simulink model "COM_BancMonitor"  (Simulink 8.6)
settings: Solver=FixedStepDiscrete  StartTime=0.0  StopTime=inf  FixedStep=ComMinSampleTime  RelTol=1e-3
values from neighbouring files (symbols this model uses):
  ComMinSampleTime = 1/400    (= 0.0025)    [init_BancMonitor.m]
  g = 9.81    [init_BancMonitor.m]
  LandingHeight = 0.08    [init_BancMonitor.m]
  Ts_AttitudeLoop = 1/200    (= 0.005)    [init_BancMonitor.m]
  Ts_PositionLoop = 1/100    (= 0.01)    [init_BancMonitor.m]
undefined symbols (not defined in the file or in its folder): a_PWM, b_PWM, BiasAcc, DiscIntNeverNeededParam, Gumstix, m, MaxThrottle, MinThrottle, MPU6050, PositionSecuMax, PositionSecuMin, Tacc, time_unfolding, Tmax, Tmin, TorquesSat, UAVstruct
undefined symbols (not defined in the file): AccMax, AccMaxScenario, AccMin, AccMinScenario, b_est0, dc_open, PositionMax, PositionMin, SpeedMax, SpeedMaxScenario, SpeedMin, SpeedMinScenario, Ts_detector, Ts_Wifi
libraries: simulink x34, custom_lib x27, simulink_extras x11
(part 3 of 3)

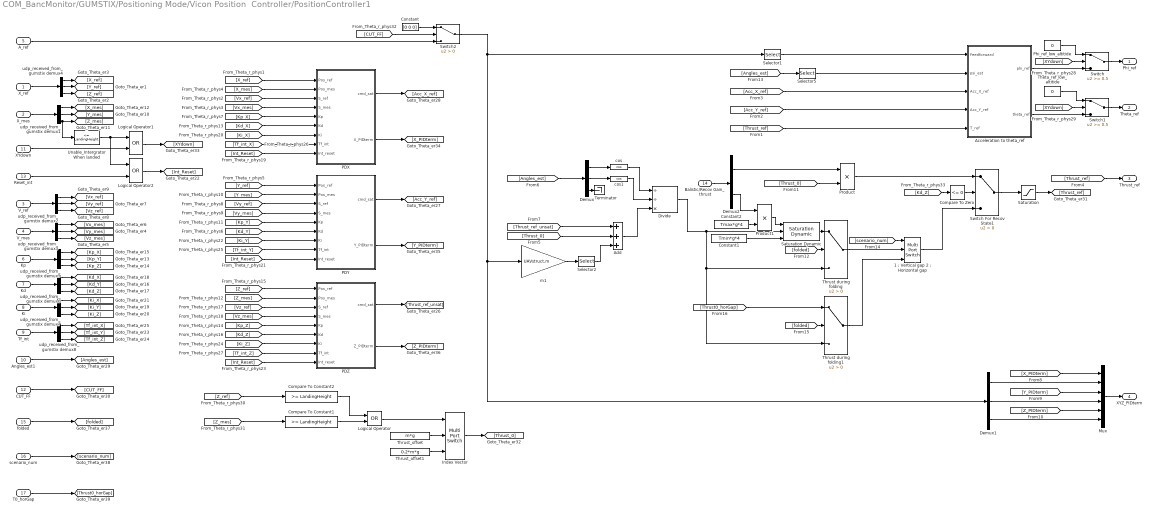
== system COM_BancMonitor/GUMSTIX/Positioning Mode/Vicon Position  Controller/PositionController1 ==
  X_ref : Inport
  X_mes : Inport  Port=2
  V_ref : Inport  Port=3
  V_mes : Inport  Port=4
  A_ref : Inport  Port=5
  Kp : Inport  Port=6
  Kd : Inport  Port=7
  Ki : Inport  Port=8
  Tf_int : Inport  Port=9
  Angles_est1 : Inport  Port=10
  XYdown : Inport  Port=11
  CUT_FF : Inport  Port=12
  Reset_int : Inport  Port=13
  Balistic/Recov Gain_thrust : Inport  Port=14
  folded : Inport  Port=15
  scenario_num : Inport  Port=16
  T0_horGap : Inport  Port=17
  "1 : Vertical gap 2 : Horizontal gap" : MultiPortSwitch  Inputs=2
  Acceleration to theta_ref : Subsystem
  Add : Sum  Inputs=+++
  Compare To Constant1 : simulink/Logic and Bit Operations/Compare To Constant  relop=>=  const=LandingHeight  OutDataTypeStr=uint8
  Compare To Constant2 : simulink/Logic and Bit Operations/Compare To Constant  relop=>=  const=LandingHeight  OutDataTypeStr=uint8
  Compare To Zero : simulink/Logic and Bit Operations/Compare To Zero  relop=<=  OutDataTypeStr=boolean
  Constant : Constant  Value=[0 0 0]  OutDataTypeStr=Inherit: Inherit via back propagation
  Constant1 : Constant  Value=Tmin*g*4  OutDataTypeStr=Inherit: Inherit via back propagation
  Constant2 : Constant  Value=Tmax*g*4  OutDataTypeStr=Inherit: Inherit via back propagation
  Demux : Demux  Outputs=3
  Demux1 : Demux  Outputs=3
  Demux2 : Demux  Outputs=2
  Divide : Product  Inputs=//*
  Index Vector : MultiPortSwitch  Inputs=2  DiagnosticForDefault=None
  Logical Operator : Logic  Operator=OR  AllPortsSameDT=off  OutDataTypeStr=boolean
  Logical Operator1 : Logic  Operator=OR  AllPortsSameDT=off  OutDataTypeStr=boolean
  Logical Operator2 : Logic  Operator=OR  AllPortsSameDT=off  OutDataTypeStr=boolean
  Mux : Mux  Inputs=[5 1 5 1 5 1]
  PDX : Subsystem  mask{Max_Sat=20*pi/180*9.81, Min_Sat=-20*pi/180*9.81}
  PDY : Subsystem  mask{Max_Sat=20*pi/180*9.81, Min_Sat=-20*pi/180*9.81}
  PDZ : Subsystem  mask{Max_Sat=Tmax*g*4, Min_Sat=Tmin*g*4}
  Phi_ref_low_altitide : Constant  Value=0  OutDataTypeStr=Inherit: Inherit via back propagation
  Product : Product
  Product1 : Product
  Saturation : Saturate  UpperLimit=Tmax*g*4  LowerLimit=Tmin*g*4
  Saturation Dynamic : simulink/Discontinuities/Saturation Dynamic  OutMin=[]  OutMax=[]  OutDataTypeStr=Inherit: Same as second input  OutDataType=fixdt(1, 16)  OutScaling=2^-10  DoSatur=off
  Selector1 : Selector  InputPortWidth=3  IndexOptions=Index vector (dialog)  Indices=[1 2]  OutputSizes=1
  Selector2 : Selector  InputPortWidth=3  IndexOptions=Index vector (dialog)  Indices=[3]  OutputSizes=1
  Selector5 : Selector  InputPortWidth=3  IndexOptions=Index vector (dialog)  Indices=[3]  OutputSizes=1
  Switch : Switch  Threshold=0.5
  Switch For Recov State1 : Switch  Criteria=u2 > Threshold
  Switch1 : Switch  Threshold=0.5
  Switch2 : Switch  Criteria=u2 > Threshold
  Terminator : Terminator
  Theta_ref_low_altitide : Constant  Value=0  OutDataTypeStr=Inherit: Inherit via back propagation
  Thrust during folding : Switch  Criteria=u2 > Threshold
  Thrust during folding1 : Switch  Criteria=u2 > Threshold
  Thrust_offset : Constant  Value=m*g  OutDataTypeStr=single  SampleTime=-1
  Thrust_offset1 : Constant  Value=0.2*m*g  OutDataTypeStr=single  SampleTime=-1
  Unable_Intergrator When landed : simulink/Logic and Bit Operations/Compare To Constant  relop=<=  const=LandingHeight  OutDataTypeStr=uint8
  cos : Trigonometry  Operator=cos
  cos1 : Trigonometry  Operator=cos
  m1 : Gain  Gain=UAVstruct.m
  udp_received_from_gumstix demux{1..8} (8 alike) : Demux  Outputs=[1 1 1]
  Phi_ref : Outport
  Theta_ref : Outport  Port=2
  Thrust_ref : Outport  Port=3
  XYZ_PIDterm : Outport  Port=4
  wires:
  udp_received_from_gumstix demux3/3 -> [Vz_mes]
  udp_received_from_gumstix demux3/2 -> [Vy_mes]
  udp_received_from_gumstix demux3/1 -> [Vx_mes]
  V_mes/1 -> udp_received_from_gumstix demux3/1
  udp_received_from_gumstix demux4/1 -> [X_ref]
  udp_received_from_gumstix demux4/2 -> [Y_ref]
  X_mes/1 -> udp_received_from_gumstix demux1/1
  udp_received_from_gumstix demux1/1 -> [X_mes]
  udp_received_from_gumstix demux1/2 -> [Y_mes]
  udp_received_from_gumstix demux1/3 -> [Z_mes], Unable_Intergrator When landed/1
  udp_received_from_gumstix demux2/3 -> [Vz_ref]
  udp_received_from_gumstix demux2/2 -> [Vy_ref]
  udp_received_from_gumstix demux2/1 -> [Vx_ref]
  V_ref/1 -> udp_received_from_gumstix demux2/1
  Kp/1 -> udp_received_from_gumstix demux5/1
  udp_received_from_gumstix demux5/3 -> [Kp_Z]
  udp_received_from_gumstix demux5/2 -> [Kp_Y]
  udp_received_from_gumstix demux5/1 -> [Kp_X]
  Kd/1 -> udp_received_from_gumstix demux6/1
  udp_received_from_gumstix demux6/3 -> [Kd_Z]
  udp_received_from_gumstix demux6/2 -> [Kd_Y]
  udp_received_from_gumstix demux6/1 -> [Kd_X]
  udp_received_from_gumstix demux4/3 -> [Z_ref]
  udp_received_from_gumstix demux7/3 -> [Ki_Z]
  udp_received_from_gumstix demux7/2 -> [Ki_Y]
  udp_received_from_gumstix demux7/1 -> [Ki_X]
  Ki/1 -> udp_received_from_gumstix demux7/1
  udp_received_from_gumstix demux8/3 -> [Tf_int_Z]
  udp_received_from_gumstix demux8/2 -> [Tf_int_Y]
  udp_received_from_gumstix demux8/1 -> [Tf_int_X]
  Tf_int/1 -> udp_received_from_gumstix demux8/1
  Acceleration to theta_ref/1(phi_ref) -> Switch/3
  [XYdown] -> Switch/2
  [XYdown] -> Switch1/2
  Acceleration to theta_ref/2(theta_ref) -> Switch1/3
  Switch1/1 -> Theta_ref/1
  Switch/1 -> Phi_ref/1
  Phi_ref_low_altitide/1 -> Switch/1
  Theta_ref_low_altitide/1 -> Switch1/1
  [Acc_X_ref] -> Acceleration to theta_ref/3(Acc_X_ref)
  [Acc_Y_ref] -> Acceleration to theta_ref/4(Acc_Y_ref)
  [Thrust_ref] -> Thrust_ref/1
  [Thrust_ref] -> Acceleration to theta_ref/5(T_ref)
  Selector5/1 -> Acceleration to theta_ref/2(psi_est)
  [Angles_est] -> Selector5/1
  Angles_est1/1 -> [Angles_est]
  [Thrust_0] -> Add/2
  [Angles_est] -> Demux/1
  Demux/3 -> Terminator/1
  Demux/1 -> cos/1
  Demux/2 -> cos1/1
  cos/1 -> Divide/1
  cos1/1 -> Divide/2
  [Thrust_ref_unsat] -> Add/1
  Add/1 -> Divide/3
  Selector2/1 -> Add/3
  Selector1/1 -> Acceleration to theta_ref/1(Feedforward)
  Saturation/1 -> [Thrust_ref]
  X_ref/1 -> udp_received_from_gumstix demux4/1
  m1/1 -> Selector2/1
  Thrust_offset/1 -> Index Vector/2
  Thrust_offset1/1 -> Index Vector/3
  Logical Operator/1 -> Index Vector/1
  Compare To Constant1/1 -> Logical Operator/2
  Compare To Constant2/1 -> Logical Operator/1
  [Z_mes] -> Compare To Constant1/1
  [Z_ref] -> Compare To Constant2/1
  Index Vector/1 -> [Thrust_0]
  Unable_Intergrator When landed/1 -> Logical Operator2/1, Logical Operator1/1
  XYdown/1 -> Logical Operator1/2
  Logical Operator1/1 -> [XYdown]
  CUT_FF/1 -> [CUT_FF]
  [CUT_FF] -> Switch2/2
  A_ref/1 -> Switch2/3
  Switch2/1 -> Selector1/1, Demux1/1, m1/1
  Constant/1 -> Switch2/1
  Logical Operator2/1 -> [Int_Reset]
  Reset_int/1 -> Logical Operator2/2
  [X_ref] -> PDX/1(Pos_ref)
  [X_mes] -> PDX/2(Pos_mes)
  [Kp_X] -> PDX/5(Kp)
  [Kd_X] -> PDX/6(Kd)
  [Vx_mes] -> PDX/4(S_mes)
  [Y_ref] -> PDY/1(Pos_ref)
  [Y_mes] -> PDY/2(Pos_mes)
  [Kp_Y] -> PDY/5(Kp)
  [Kd_Y] -> PDY/6(Kd)
  [Vy_ref] -> PDY/3(S_ref)
  [Vy_mes] -> PDY/4(S_mes)
  [Vx_ref] -> PDX/3(S_ref)
  [Ki_X] -> PDX/7(Ki)
  [Ki_Y] -> PDY/7(Ki)
  [Int_Reset] -> PDY/9(Int_reset)
  [Z_ref] -> PDZ/1(Pos_ref)
  [Z_mes] -> PDZ/2(Pos_mes)
  [Vz_ref] -> PDZ/3(S_ref)
  [Vz_mes] -> PDZ/4(S_mes)
  [Kp_Z] -> PDZ/5(Kp)
  [Kd_Z] -> PDZ/6(Kd)
  [Ki_Z] -> PDZ/7(Ki)
  [Tf_int_Y] -> PDY/8(Tf_int)
  [Tf_int_X] -> PDX/8(Tf_int)
  [Int_Reset] -> PDX/9(Int_reset)
  [Tf_int_Z] -> PDZ/8(Tf_int)
  [Int_Reset] -> PDZ/9(Int_reset)
  PDY/1(cmd_sat) -> [Acc_Y_ref]
  PDX/1(cmd_sat) -> [Acc_X_ref]
  PDZ/1(cmd_sat) -> [Thrust_ref_unsat]
  PDX/2(X_PIDterm) -> [X_PIDterm]
  PDY/2(Y_PIDterm) -> [Y_PIDterm]
  PDZ/2(Z_PIDterm) -> [Z_PIDterm]
  [Y_PIDterm] -> Mux/3
  Mux/1 -> XYZ_PIDterm/1
  [X_PIDterm] -> Mux/1
  [Z_PIDterm] -> Mux/5
  [Kd_Z] -> Compare To Zero/1
  Compare To Zero/1 -> Switch For Recov State1/2
  Switch For Recov State1/1 -> Saturation/1
  [Thrust_0] -> Product/2
  Product/1 -> Switch For Recov State1/1
  Demux1/1 -> Mux/2
  Demux1/2 -> Mux/4
  Demux1/3 -> Mux/6
  folded/1 -> [folded]
  [folded] -> Thrust during folding/2
  Saturation Dynamic/1 -> Thrust during folding/1
  Divide/1 -> Saturation Dynamic/2, Thrust during folding1/3, Thrust during folding/3
  Constant1/1 -> Saturation Dynamic/3
  Product1/1 -> Saturation Dynamic/1
  Constant2/1 -> Product1/2
  Balistic/Recov Gain_thrust/1 -> Demux2/1
  Demux2/1 -> Product/1
  Demux2/2 -> Product1/1
  scenario_num/1 -> [scenario_num]
  Thrust during folding/1 -> "1 : Vertical gap 2 : Horizontal gap"/2
  [folded] -> Thrust during folding1/2
  "1 : Vertical gap 2 : Horizontal gap"/1 -> Switch For Recov State1/3
  T0_horGap/1 -> [Thrust0_horGap]
  [Thrust0_horGap] -> Thrust during folding1/1
  Thrust during folding1/1 -> "1 : Vertical gap 2 : Horizontal gap"/3
  [scenario_num] -> "1 : Vertical gap 2 : Horizontal gap"/1

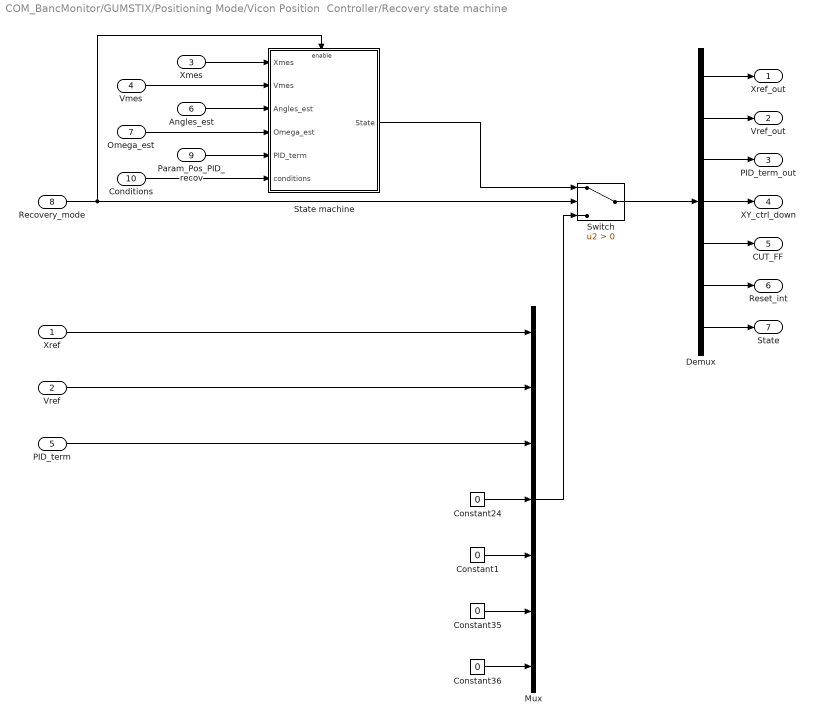
== system COM_BancMonitor/GUMSTIX/Positioning Mode/Vicon Position  Controller/Recovery state machine ==
  Xref : Inport
  Vref : Inport  Port=2
  Xmes : Inport  Port=3
  Vmes : Inport  Port=4
  PID_term : Inport  Port=5
  Angles_est : Inport  Port=6
  Omega_est : Inport  Port=7
  Recovery_mode : Inport  Port=8
  Param_Pos_PID_recov : Inport  Port=9
  Conditions : Inport  Port=10
  Constant{1,24,35..36} (4 alike) : Constant  Value=0  OutDataTypeStr=Inherit: Inherit via back propagation
  Demux : Demux  Outputs=[3 3 12 1 1 1 1]
  Mux : Mux  Inputs=7
  State machine : Subsystem
  Switch : Switch  Criteria=u2 > Threshold
  Xref_out : Outport
  Vref_out : Outport  Port=2
  PID_term_out : Outport  Port=3
  XY_ctrl_down : Outport  Port=4
  CUT_FF : Outport  Port=5
  Reset_int : Outport  Port=6
  State : Outport  Port=7
  wires:
  Demux/1 -> Xref_out/1
  Demux/2 -> Vref_out/1
  Demux/3 -> PID_term_out/1
  Demux/4 -> XY_ctrl_down/1
  Demux/5 -> CUT_FF/1
  Xref/1 -> Mux/1
  Vref/1 -> Mux/2
  Constant24/1 -> Mux/4
  Constant1/1 -> Mux/5
  Mux/1 -> Switch/3
  Vmes/1 -> State machine/2(Vmes)
  Demux/6 -> Reset_int/1
  Constant35/1 -> Mux/6
  PID_term/1 -> Mux/3
  Switch/1 -> Demux/1
  Demux/7 -> State/1
  Constant36/1 -> Mux/7
  Recovery_mode/1 -> Switch/2, State machine/Enable
  State machine/1(State) -> Switch/1
  Angles_est/1 -> State machine/3(Angles_est)
  Omega_est/1 -> State machine/4(Omega_est)
  Xmes/1 -> State machine/1(Xmes)
  Conditions/1 -> State machine/6(conditions)
  Param_Pos_PID_recov/1 -> State machine/5(PID_term)

== system COM_BancMonitor/GUMSTIX/Attitude controller/CTL_ATT_NL/Angles Disturbances/Triggered Subsystem ==
  AnglesDist Mag : Inport
  Dt : Inport  Port=2
  Enable : EnablePort  StatesWhenEnabling=reset
  Constant : Constant  OutDataTypeStr=single
  Discrete-Time Integrator : DiscreteIntegrator  SampleTime=-1  ICPrevOutput=DiscIntNeverNeededParam  ICPrevScaledInput=DiscIntNeverNeededParam
  MATLAB Function : MATLAB Function  TreatAsAtomicUnit=on
  DisturbAngles : Outport  InitialOutput=[0 0 0]
  wires:
  AnglesDist Mag/1 -> MATLAB Function/1(AnglesDistMag)
  Constant/1 -> Discrete-Time Integrator/1
  Discrete-Time Integrator/1 -> MATLAB Function/2(Time)
  Dt/1 -> MATLAB Function/3(Dt)
  MATLAB Function/1(AnglesDist) -> DisturbAngles/1

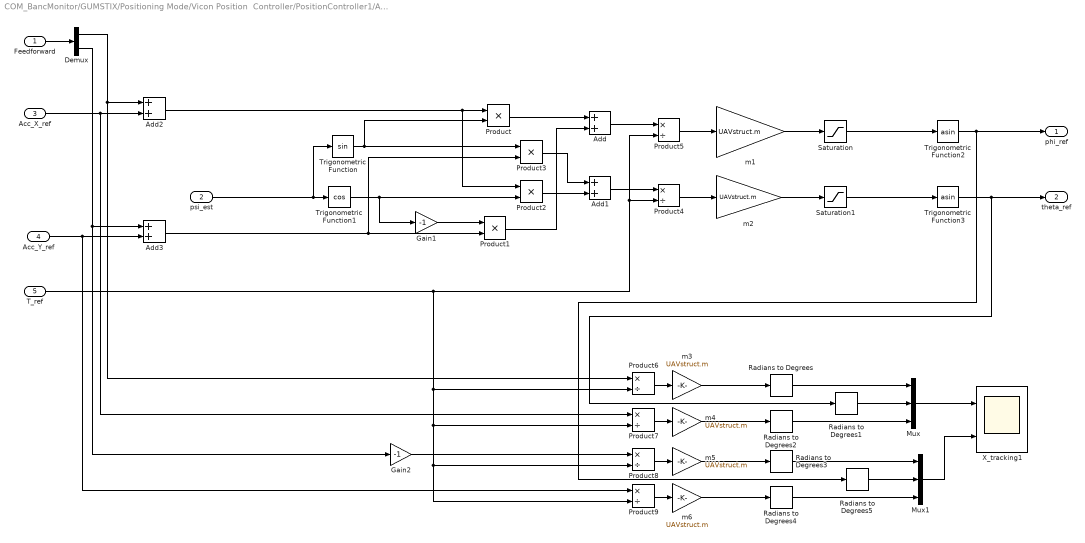
== system COM_BancMonitor/GUMSTIX/Positioning Mode/Vicon Position  Controller/PositionController1/Acceleration to theta_ref ==
  Feedforward : Inport
  psi_est : Inport  Port=2
  Acc_X_ref : Inport  Port=3
  Acc_Y_ref : Inport  Port=4
  T_ref : Inport  Port=5
  Add{,1..3} (4 alike) : Sum
  Demux : Demux  Outputs=2
  Gain1 : Gain  Gain=-1
  Gain2 : Gain  Gain=-1
  Mux : Mux  Inputs=3
  Mux1 : Mux  Inputs=3
  Product{,1..3} (4 alike) : Product  RndMeth=Zero
  Product{4..9} (6 alike) : Product  Inputs=*/  RndMeth=Zero
  Radians to Degrees{,1..5} (6 alike) : simulink_extras/Transformations/Radians to Degrees
  Saturation : Saturate  UpperLimit=sin(45*pi/180)  LowerLimit=sin(-45*pi/180)
  Saturation1 : Saturate  UpperLimit=sin(45*pi/180)  LowerLimit=sin(-45*pi/180)
  Trigonometric Function : Trigonometry
  Trigonometric Function1 : Trigonometry  Operator=cos
  Trigonometric Function2 : Trigonometry  Operator=asin
  Trigonometric Function3 : Trigonometry  Operator=asin
  X_tracking1 : Scope  NumInputPorts=2
  m{1..6} (6 alike) : Gain  Gain=UAVstruct.m
  phi_ref : Outport
  theta_ref : Outport  Port=2
  wires:
  psi_est/1 -> Trigonometric Function/1, Trigonometric Function1/1
  Trigonometric Function/1 -> Product3/1, Product/2
  Trigonometric Function1/1 -> Product2/2, Gain1/1
  Product1/1 -> Add/2
  Product/1 -> Add/1
  Product3/1 -> Add1/1
  Product2/1 -> Add1/2
  Acc_X_ref/1 -> Add2/2, Product7/1
  Demux/1 -> Add2/1, Product6/1
  Demux/2 -> Add3/1, Gain2/1
  Acc_Y_ref/1 -> Add3/2, Product9/1
  Add2/1 -> Product2/1, Product/1
  Add3/1 -> Product3/2, Product1/2
  Product5/1 -> m1/1
  m1/1 -> Saturation/1
  Add/1 -> Product5/1
  Trigonometric Function2/1 -> phi_ref/1, Radians to Degrees5/1
  Product4/1 -> m2/1
  m2/1 -> Saturation1/1
  Trigonometric Function3/1 -> theta_ref/1, Radians to Degrees1/1
  Add1/1 -> Product4/1
  T_ref/1 -> Product4/2, Product5/2, Product6/2, Product7/2, Product8/2, Product9/2
  Saturation/1 -> Trigonometric Function2/1
  Saturation1/1 -> Trigonometric Function3/1
  Gain1/1 -> Product1/1
  Radians to Degrees/1 -> Mux/1
  Radians to Degrees1/1 -> Mux/2
  Product6/1 -> m3/1
  m3/1 -> Radians to Degrees/1
  Product7/1 -> m4/1
  m4/1 -> Radians to Degrees2/1
  Radians to Degrees2/1 -> Mux/3
  Mux/1 -> X_tracking1/1
  Mux1/1 -> X_tracking1/2
  Product8/1 -> m5/1
  m5/1 -> Radians to Degrees3/1
  Radians to Degrees3/1 -> Mux1/1
  Radians to Degrees4/1 -> Mux1/3
  Product9/1 -> m6/1
  m6/1 -> Radians to Degrees4/1
  Radians to Degrees5/1 -> Mux1/2
  Gain2/1 -> Product8/1
  Feedforward/1 -> Demux/1

== system COM_BancMonitor/GUMSTIX/Positioning Mode/Vicon Position  Controller/PositionController1/PDX ==
  Pos_ref : Inport
  Pos_mes : Inport  Port=2
  S_ref : Inport  Port=3
  S_mes : Inport  Port=4
  Kp : Inport  Port=5
  Kd : Inport  Port=6
  Ki : Inport  Port=7
  Tf_int : Inport  Port=8
  Int_reset : Inport  Port=9
  Add : Sum  Inputs=+++
  Add1 : Sum  Inputs=+-
  Add2 : Sum  Inputs=+-
  Discrete filter first_ordrer1 : Subsystem
  Discrete-Time Integrator1 : DiscreteIntegrator  ExternalReset=level  SampleTime=-1  LimitOutput=on  UpperSaturationLimit=Max_Sat  LowerSaturationLimit=Min_Sat  ICPrevOutput=DiscIntNeverNeededParam  ICPrevScaledInput=DiscIntNeverNeededParam
  Mux : Mux  Inputs=5
  Product : Product  RndMeth=Zero
  Product1 : Product  RndMeth=Zero
  Product2 : Product  RndMeth=Zero
  cmd_sat : Outport
  X_PIDterm : Outport  Port=2
  wires:
  Tf_int/1 -> Discrete filter first_ordrer1/2(z0)
  Discrete filter first_ordrer1/1(y) -> Discrete-Time Integrator1/1
  Product1/1 -> Discrete filter first_ordrer1/1(u)
  Pos_mes/1 -> Add2/2
  Add2/1 -> Mux/1, Product/1
  Pos_ref/1 -> Add2/1
  Kp/1 -> Product/2
  Product/1 -> Mux/3, Add/1, Product1/1
  Kd/1 -> Product2/2
  S_ref/1 -> Add1/1
  S_mes/1 -> Add1/2
  Add1/1 -> Mux/2, Product2/1
  Product2/1 -> Mux/5, Add/3
  Ki/1 -> Product1/2
  Discrete-Time Integrator1/1 -> Mux/4, Add/2
  Int_reset/1 -> Discrete-Time Integrator1/2
  Add/1 -> cmd_sat/1
  Mux/1 -> X_PIDterm/1

== system COM_BancMonitor/GUMSTIX/Positioning Mode/Vicon Position  Controller/PositionController1/PDY ==
  Pos_ref : Inport
  Pos_mes : Inport  Port=2
  S_ref : Inport  Port=3
  S_mes : Inport  Port=4
  Kp : Inport  Port=5
  Kd : Inport  Port=6
  Ki : Inport  Port=7
  Tf_int : Inport  Port=8
  Int_reset : Inport  Port=9
  Add : Sum  Inputs=+++
  Add1 : Sum  Inputs=+-
  Add2 : Sum  Inputs=+-
  Discrete filter first_ordrer1 : Subsystem
  Discrete-Time Integrator1 : DiscreteIntegrator  ExternalReset=level  SampleTime=-1  LimitOutput=on  UpperSaturationLimit=Max_Sat  LowerSaturationLimit=Min_Sat  ICPrevOutput=DiscIntNeverNeededParam  ICPrevScaledInput=DiscIntNeverNeededParam
  Mux : Mux  Inputs=5
  Product : Product  RndMeth=Zero
  Product1 : Product  RndMeth=Zero
  Product2 : Product  RndMeth=Zero
  cmd_sat : Outport
  Y_PIDterm : Outport  Port=2
  wires:
  Int_reset/1 -> Discrete-Time Integrator1/2
  Ki/1 -> Product1/2
  Add1/1 -> Mux/2, Product2/1
  S_mes/1 -> Add1/2
  S_ref/1 -> Add1/1
  Kd/1 -> Product2/2
  Kp/1 -> Product/2
  Pos_ref/1 -> Add2/1
  Add2/1 -> Mux/1, Product/1
  Pos_mes/1 -> Add2/2
  Product1/1 -> Discrete filter first_ordrer1/1(u)
  Discrete filter first_ordrer1/1(y) -> Discrete-Time Integrator1/1
  Tf_int/1 -> Discrete filter first_ordrer1/2(z0)
  Add/1 -> cmd_sat/1
  Product/1 -> Mux/3, Product1/1, Add/1
  Product2/1 -> Mux/5, Add/3
  Discrete-Time Integrator1/1 -> Mux/4, Add/2
  Mux/1 -> Y_PIDterm/1

== system COM_BancMonitor/GUMSTIX/Positioning Mode/Vicon Position  Controller/PositionController1/PDZ ==
  Pos_ref : Inport
  Pos_mes : Inport  Port=2
  S_ref : Inport  Port=3
  S_mes : Inport  Port=4
  Kp : Inport  Port=5
  Kd : Inport  Port=6
  Ki : Inport  Port=7
  Tf_int : Inport  Port=8
  Int_reset : Inport  Port=9
  Add : Sum  Inputs=+++
  Add1 : Sum  Inputs=+-
  Add2 : Sum  Inputs=+-
  Discrete filter first_ordrer1 : Subsystem
  Discrete-Time Integrator1 : DiscreteIntegrator  ExternalReset=level  SampleTime=-1  LimitOutput=on  UpperSaturationLimit=Max_Sat*0.5  LowerSaturationLimit=-Max_Sat*0.5  ICPrevOutput=DiscIntNeverNeededParam  ICPrevScaledInput=DiscIntNeverNeededParam
  Mux : Mux  Inputs=5
  Product : Product  RndMeth=Zero
  Product1 : Product  RndMeth=Zero
  Product2 : Product  RndMeth=Zero
  cmd_sat : Outport
  Z_PIDterm : Outport  Port=2
  wires:
  Pos_mes/1 -> Add2/2
  Add2/1 -> Mux/1, Product/1
  Pos_ref/1 -> Add2/1
  Kp/1 -> Product/2
  Kd/1 -> Product2/2
  S_ref/1 -> Add1/1
  S_mes/1 -> Add1/2
  Add1/1 -> Mux/2, Product2/1
  Ki/1 -> Product1/2
  Int_reset/1 -> Discrete-Time Integrator1/2
  Tf_int/1 -> Discrete filter first_ordrer1/2(z0)
  Discrete filter first_ordrer1/1(y) -> Discrete-Time Integrator1/1
  Product1/1 -> Discrete filter first_ordrer1/1(u)
  Add/1 -> cmd_sat/1
  Product/1 -> Mux/3, Product1/1, Add/1
  Product2/1 -> Mux/5, Add/3
  Discrete-Time Integrator1/1 -> Mux/4, Add/2
  Mux/1 -> Z_PIDterm/1

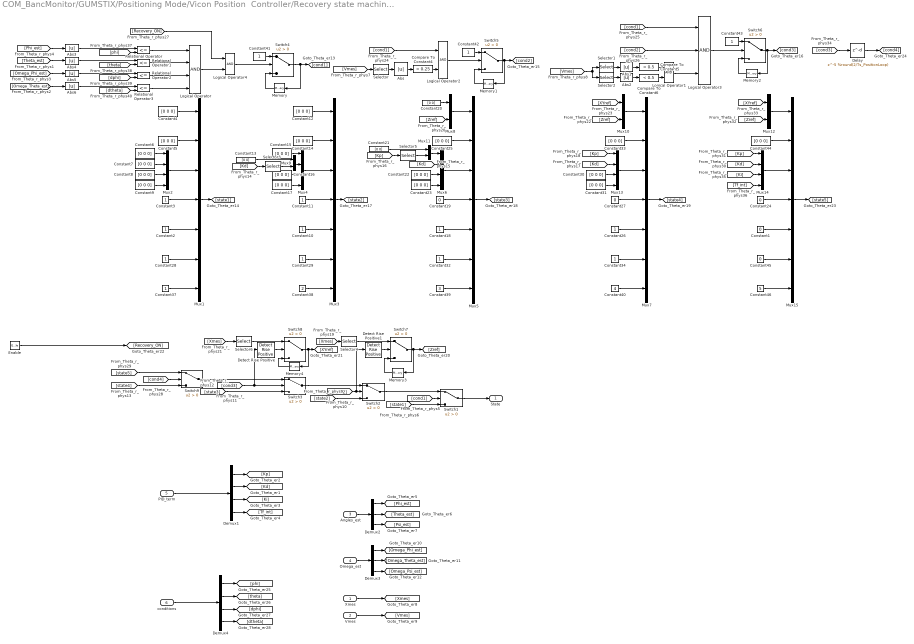
== system COM_BancMonitor/GUMSTIX/Positioning Mode/Vicon Position  Controller/Recovery state machine/State machine ==
  Xmes : Inport
  Vmes : Inport  Port=2
  Angles_est : Inport  Port=3
  Omega_est : Inport  Port=4
  PID_term : Inport  Port=5
  conditions : Inport  Port=6
  Enable : EnablePort  StatesWhenEnabling=reset  ShowOutputPort=on
  Abs{,1..6} (7 alike) : Abs
  Compare To Constant4 : simulink/Logic and Bit Operations/Compare To Constant  relop=<  const=0.25  OutDataTypeStr=boolean
  Compare To Constant5 : simulink/Logic and Bit Operations/Compare To Constant  relop=<  const=0.5  OutDataTypeStr=boolean
  Compare To Constant6 : simulink/Logic and Bit Operations/Compare To Constant  relop=<  const=0.5  OutDataTypeStr=boolean
  Constant{1,19,24,27,45} (5 alike) : Constant  Value=0  OutDataTypeStr=Inherit: Inherit via back propagation
  Constant{2..3,10..11,18,26,28..29,32,34,37,41..43} (14 alike) : Constant  OutDataTypeStr=Inherit: Inherit via back propagation
  Constant{4..9,12,14..17,22..23,25,30..31,33,44} (18 alike) : Constant  Value=[0 0 0]  OutDataTypeStr=Inherit: Inherit via back propagation
  Constant13 : Constant  Value=[0 0]  OutDataTypeStr=Inherit: Inherit via back propagation
  Constant20 : Constant  Value=[0 0]  OutDataTypeStr=Inherit: Inherit via back propagation
  Constant21 : Constant  Value=[0 0]  OutDataTypeStr=Inherit: Inherit via back propagation
  Constant38 : Constant  Value=2  OutDataTypeStr=Inherit: Inherit via back propagation
  Constant39 : Constant  Value=3  OutDataTypeStr=Inherit: Inherit via back propagation
  Constant40 : Constant  Value=4  OutDataTypeStr=Inherit: Inherit via back propagation
  Constant46 : Constant  Value=5  OutDataTypeStr=Inherit: Inherit via back propagation
  Delay : Delay  DelayLength=5 %round(2/Ts_PositionLoop)  InitialCondition=0  SampleTime=Ts_PositionLoop
  Demux1 : Demux
  Demux2 : Demux  Outputs=3
  Demux3 : Demux  Outputs=3
  Demux4 : Demux
  Detect Rise Positive : simulink/Logic and Bit Operations/Detect Rise Positive  vinit=0  InputProcessing=Inherited  OutDataTypeStr=boolean
  Detect Rise Positive1 : simulink/Logic and Bit Operations/Detect Rise Positive  vinit=0  InputProcessing=Inherited  OutDataTypeStr=boolean
  Logical Operator : Logic  Inputs=4  AllPortsSameDT=off  OutDataTypeStr=boolean
  Logical Operator1 : Logic  AllPortsSameDT=off  OutDataTypeStr=boolean
  Logical Operator2 : Logic  AllPortsSameDT=off  OutDataTypeStr=boolean
  Logical Operator3 : Logic  Inputs=3  AllPortsSameDT=off  OutDataTypeStr=boolean
  Logical Operator4 : Logic  AllPortsSameDT=off  OutDataTypeStr=boolean
  Memory{,1..4} (5 alike) : Memory  InheritSampleTime=on
  Mux{1,3,5,7,15} (5 alike) : Mux  Inputs=7
  Mux{8..12} (5 alike) : Mux  Inputs=2
  Mux{2,4,6,13..14} (5 alike) : Mux
  Relational Operator{,1..3} (4 alike) : RelationalOperator  Operator=<=  OutDataTypeStr=boolean
  Selector{,3..5} (4 alike) : Selector  InputPortWidth=3  IndexOptions=Index vector (dialog)  Indices=[3]  OutputSizes=1
  Selector1 : Selector  InputPortWidth=3  IndexOptions=Index vector (dialog)  Indices=[1]  OutputSizes=1
  Selector2 : Selector  InputPortWidth=3  IndexOptions=Index vector (dialog)  Indices=[2]  OutputSizes=1
  Selector6 : Selector  InputPortWidth=3  IndexOptions=Index vector (dialog)  Indices=[1 2]  OutputSizes=1
  Switch{1..9} (9 alike) : Switch  Criteria=u2 > Threshold
  State : Outport  OutputWhenDisabled=reset  InitialOutput=1
  wires:
  Mux2/1 -> Mux1/3
  Constant2/1 -> Mux1/5
  Constant3/1 -> Mux1/4
  Constant6/1 -> Mux2/1
  Constant7/1 -> Mux2/2
  Constant8/1 -> Mux2/3
  Constant9/1 -> Mux2/4
  Constant4/1 -> Mux1/1
  Constant5/1 -> Mux1/2
  [Phi_est] -> Abs3/1
  [Theta_est] -> Abs4/1
  [Omega_Phi_est] -> Abs5/1
  [Omega_Theta_est] -> Abs6/1
  Relational Operator/1 -> Logical Operator/1
  Relational Operator1/1 -> Logical Operator/2
  Relational Operator2/1 -> Logical Operator/3
  Relational Operator3/1 -> Logical Operator/4
  [cond1] -> Switch1/2
  Mux1/1 -> [state1]
  [state1] -> Switch1/3
  Switch1/1 -> State/1
  [Vmes] -> Selector/1
  Selector/1 -> Abs/1
  Abs/1 -> Compare To Constant4/1
  [Vmes] -> Selector1/1, Selector2/1
  Selector2/1 -> Abs2/1
  Compare To Constant5/1 -> Logical Operator1/1
  Compare To Constant6/1 -> Logical Operator1/2
  Selector1/1 -> Abs1/1
  Abs1/1 -> Compare To Constant5/1
  Abs2/1 -> Compare To Constant6/1
  [cond2] -> Detect Rise Positive1/1, Switch2/2
  Switch2/1 -> Switch1/1
  [state2] -> Switch2/3
  [cond3] -> Detect Rise Positive/1, Switch3/2
  [state3] -> Switch3/3
  Switch3/1 -> Switch2/1
  Switch9/1 -> Switch3/1
  Mux4/1 -> Mux3/3
  Constant10/1 -> Mux3/5
  Constant11/1 -> Mux3/4
  Constant15/1 -> Mux4/1
  Mux9/1 -> Mux4/2
  Constant16/1 -> Mux4/3
  Constant17/1 -> Mux4/4
  Constant12/1 -> Mux3/1
  Constant14/1 -> Mux3/2
  Mux3/1 -> [state2]
  Constant18/1 -> Mux5/5
  Constant19/1 -> Mux5/4
  Constant25/1 -> Mux5/2
  Mux5/1 -> [state3]
  Constant26/1 -> Mux7/5
  Constant27/1 -> Mux7/4
  Constant33/1 -> Mux7/2
  Mux7/1 -> [state4]
  [Kd] -> Selector3/1
  Constant13/1 -> Mux9/1
  Selector3/1 -> Mux9/2
  Mux6/1 -> Mux5/3
  Mux11/1 -> Mux6/1
  [Kd] -> Mux6/2
  Constant22/1 -> Mux6/3
  Constant23/1 -> Mux6/4
  [Kp] -> Selector5/1
  Constant21/1 -> Mux11/1
  Selector5/1 -> Mux11/2
  Mux13/1 -> Mux7/3
  [Kp] -> Mux13/1
  [Kd] -> Mux13/2
  Constant30/1 -> Mux13/3
  Constant31/1 -> Mux13/4
  Mux8/1 -> Mux5/1
  Constant20/1 -> Mux8/1
  [Xmes] -> Selector4/1
  [Zref] -> Mux8/2
  Switch8/1 -> Memory4/1, [XYref]
  [Xmes] -> Selector6/1
  Mux10/1 -> Mux7/1
  [XYref] -> Mux10/1
  [Zref] -> Mux10/2
  Constant28/1 -> Mux1/6
  Constant29/1 -> Mux3/6
  Constant32/1 -> Mux5/6
  Constant34/1 -> Mux7/6
  Compare To Constant4/1 -> Logical Operator2/2
  Logical Operator1/1 -> Logical Operator3/3
  [cond1] -> Logical Operator3/1
  Abs5/1 -> Relational Operator2/1
  Abs6/1 -> Relational Operator3/1
  Constant37/1 -> Mux1/7
  Constant38/1 -> Mux3/7
  Constant39/1 -> Mux5/7
  Constant40/1 -> Mux7/7
  Logical Operator/1 -> Logical Operator4/2
  Memory1/1 -> Switch5/3
  Switch5/1 -> [cond2], Memory1/1
  Logical Operator2/1 -> Switch5/2
  Constant42/1 -> Switch5/1
  Memory2/1 -> Switch6/3
  Switch6/1 -> [cond3], Memory2/1
  Logical Operator3/1 -> Switch6/2
  Constant43/1 -> Switch6/1
  Memory3/1 -> Switch7/3
  Switch7/1 -> [Zref], Memory3/1
  Selector4/1 -> Switch7/1
  Memory4/1 -> Switch8/3
  Selector6/1 -> Switch8/1
  Detect Rise Positive/1 -> Switch8/2
  Detect Rise Positive1/1 -> Switch7/2
  Demux1/1 -> [Kp]
  Demux1/2 -> [Kd]
  Demux1/3 -> [Ki]
  Demux1/4 -> [Tf_int]
  PID_term/1 -> Demux1/1
  Angles_est/1 -> Demux2/1
  Demux2/1 -> [Phi_est]
  Demux2/2 -> [Theta_est]
  Demux2/3 -> [Psi_est]
  Xmes/1 -> [Xmes]
  Vmes/1 -> [Vmes]
  Omega_est/1 -> Demux3/1
  Demux3/1 -> [Omega_Phi_est]
  Demux3/2 -> [Omega_Theta_est]
  Demux3/3 -> [Omega_Psi_est]
  Enable/1 -> [Recovery_ON]
  [cond1] -> Logical Operator2/1
  [Recovery_ON] -> Logical Operator4/1
  [cond2] -> Logical Operator3/2
  Memory/1 -> Switch4/3
  Logical Operator4/1 -> Switch4/2
  Constant41/1 -> Switch4/1
  Switch4/1 -> Memory/1, [cond1]
  [state4] -> Switch9/3
  [cond4] -> Switch9/2
  [state5] -> Switch9/1
  Constant1/1 -> Mux15/5
  Constant24/1 -> Mux15/4
  Constant44/1 -> Mux15/2
  Mux15/1 -> [state5]
  Mux14/1 -> Mux15/3
  [Kp] -> Mux14/1
  [Kd] -> Mux14/2
  [Ki] -> Mux14/3
  [Tf_int] -> Mux14/4
  Mux12/1 -> Mux15/1
  [XYref] -> Mux12/1
  [Zref] -> Mux12/2
  Constant45/1 -> Mux15/6
  Constant46/1 -> Mux15/7
  [cond3] -> Delay/1
  Delay/1 -> [cond4]
  conditions/1 -> Demux4/1
  Demux4/1 -> [phi]
  Demux4/2 -> [theta]
  Demux4/3 -> [dphi]
  Demux4/4 -> [dtheta]
  Abs3/1 -> Relational Operator/1
  [phi] -> Relational Operator/2
  [theta] -> Relational Operator1/2
  Abs4/1 -> Relational Operator1/1
  [dphi] -> Relational Operator2/2
  [dtheta] -> Relational Operator3/2

== system COM_BancMonitor/GUMSTIX/Positioning Mode/Vicon Position  Controller/PositionController1/PDX/Discrete filter first_ordrer1 ==
  u : Inport
  z0 : Inport  Port=2
  Add : Sum  Inputs=+-
  Add1 : Sum
  Constant : Constant  OutDataTypeStr=Inherit: Inherit via back propagation
  Divide : Product  Inputs=**
  Divide1 : Product  Inputs=**
  Memory : Memory  InheritSampleTime=on
  y : Outport
  wires:
  Constant/1 -> Add/1
  z0/1 -> Add/2, Divide/1
  Memory/1 -> Divide/2
  Add/1 -> Divide1/2
  u/1 -> Divide1/1
  Add1/1 -> Memory/1, y/1
  Divide1/1 -> Add1/1
  Divide/1 -> Add1/2

== system COM_BancMonitor/GUMSTIX/Positioning Mode/Vicon Position  Controller/PositionController1/PDY/Discrete filter first_ordrer1 ==
  u : Inport
  z0 : Inport  Port=2
  Add : Sum  Inputs=+-
  Add1 : Sum
  Constant : Constant  OutDataTypeStr=Inherit: Inherit via back propagation
  Divide : Product  Inputs=**
  Divide1 : Product  Inputs=**
  Memory : Memory  InheritSampleTime=on
  y : Outport
  wires:
  Divide/1 -> Add1/2
  Divide1/1 -> Add1/1
  Add1/1 -> y/1, Memory/1
  u/1 -> Divide1/1
  Add/1 -> Divide1/2
  Memory/1 -> Divide/2
  z0/1 -> Divide/1, Add/2
  Constant/1 -> Add/1

== system COM_BancMonitor/GUMSTIX/Positioning Mode/Vicon Position  Controller/PositionController1/PDZ/Discrete filter first_ordrer1 ==
  u : Inport
  z0 : Inport  Port=2
  Add : Sum  Inputs=+-
  Add1 : Sum
  Constant : Constant  OutDataTypeStr=Inherit: Inherit via back propagation
  Divide : Product  Inputs=**
  Divide1 : Product  Inputs=**
  Memory : Memory  InheritSampleTime=on
  y : Outport
  wires:
  Divide/1 -> Add1/2
  Divide1/1 -> Add1/1
  Add1/1 -> y/1, Memory/1
  u/1 -> Divide1/1
  Add/1 -> Divide1/2
  Memory/1 -> Divide/2
  z0/1 -> Divide/1, Add/2
  Constant/1 -> Add/1

== matlab function GUMSTIX/ESTIMATOR/Complementary Filter Quaternion gyro, acc, vicon GUMSTIX/Attitude_Est ==
  data: Q_hat_prec input single size=[4,1]; b_hat_prec input single size=[3,1]; gyro_imu input single size=[3,1]; acc_imu input single size=[3,1]; Q_Vicon input single size=[4,1]; dt input single size=1; k_a input single size=3; Q_hat output single size=[4,1]; b_hat output single size=[3,1]; Omega_hat output single size=[3, 1]; k_v input single size=3; k_b input single size=3; acc_ref input single size=3
function [Q_hat, b_hat, Omega_hat] = estimate_Complementary_Filter(Q_hat_prec, b_hat_prec, gyro_imu, acc_imu, Q_Vicon, dt, k_a, k_v, k_b, acc_ref)
    
    %#codegen
    
    
    % calculate the skew symetric matrix of the debiased gyro data
    Omega_hat = gyro_imu-b_hat_prec;
    
    % calculate the weighted correction 
    Q_tilde = QuaternionProduct(InvQuaternion(Q_Vicon), Q_hat_prec);
    s_tilde = Q_tilde(1);
    v_tilde = Q_tilde(2:4);
    
    alpha =    1/(norm(acc_ref)^2)*k_a.*cross(QuaternionVectorProduct(InvQuaternion(Q_hat_prec), acc_ref), acc_imu)...
             + k_v.*(s_tilde*v_tilde);
    
    % Construct the correction quaternion
    Q_corr = [        0        ;...
              Omega_hat - alpha];
    
    % determine the derivative of the rotation matrix
    dQ_hat = 0.5*QuaternionProduct(Q_hat_prec, Q_corr);
    % determine the derivative of the gyro's bias
    db_hat =k_b.*alpha;
    
    % First order Euler integration
    Q_hat = Q_hat_prec + dQ_hat*dt;
    
    % projection of the corrected quaternion (updated estimation of
    % attitude) onto Q
    Q_hat = UnitQuaternion(Q_hat);
    
    % time integration of the rotation matrix (euler forward)
    b_hat = b_hat_prec + db_hat*dt;
    
end

== matlab function GUMSTIX/Attitude controller/CTL_ATT_NL/Quaternion 2 Euler ==
  data: Q_hat input double; phi_hat output double; theta_hat output double; psi_hat output double
function [phi_hat, theta_hat, psi_hat] = rot2rad(Q_hat)
    
    %#codegen
    
    [phi_hat, theta_hat, psi_hat] = Quaternion2Euler(Q_hat);

end

== matlab function GUMSTIX/ESTIMATOR/MakeAngleContinous ==
  data: PsiEst input single; PsiCorr output single; PsiEst_prec input single; Offset_prec input single; Offset output single
function [PsiCorr, Offset] = MakeAngleContinous(PsiEst, PsiEst_prec, Offset_prec)
    %#codegen

    if(PsiEst_prec-PsiEst > pi)
        Offset = Offset_prec+2*pi;
        
    elseif (PsiEst_prec-PsiEst < -pi)
        Offset = Offset_prec-2*pi;
    else
        Offset = Offset_prec;   % do nothing
    end
    PsiCorr = PsiEst + Offset;
    
end

== matlab function GUMSTIX/Torques Disturbances/Triggered Subsystem/MATLAB Function ==
  data: TorquesDistMag input single; TorquesDist output single; Time input single; Dt input single
function TorquesDist = fcn(TorquesDistMag, Time, Dt)

    %#codegen
    
    TorquesDist = single(zeros(3,1));

    t1 = single(1);
    t2 = single(5);
    t3 = single(9);
    
    Dt = Dt/2;

    if (Time>=t1 && Time<t1+Dt)
        TorquesDist(1) = TorquesDistMag(1);
    elseif (Time>=t1+Dt && Time<t1+2*Dt)
        TorquesDist(1) = -TorquesDistMag(1);
    elseif (Time>=t2 && Time<t2+Dt)
        TorquesDist(2) = TorquesDistMag(2);
    elseif (Time>=t2+Dt && Time<t2+2*Dt)
        TorquesDist(2) = -TorquesDistMag(2);
    elseif (Time>=t3 && Time<t3+Dt)
        TorquesDist(3) = TorquesDistMag(3);
    elseif (Time>=t3+Dt && Time<t3+2*Dt)
        TorquesDist(3) = -TorquesDistMag(3);
    else
        % do nothing, all torques are null
    end

end

== matlab function GUMSTIX/Attitude controller/CTL_ATT_NL/AttCtrl Perso ==
  data: Q_ref input double size=[4, 1]; Torques output double size=[3, 1]; eR output double; Omega_ref output single size=[3,1]; Iterm output double; Dterm output double; Q_est input double size=[4, 1]; Omega_est input double size=[3, 1]; I input double size=[3, 3]; Komega_perso input double size=[3, 1]; Ktorques_perso input double size=[3, 1]; Kint_perso input double; dt input double; Pos input double; GyroTerm output double size=[3,1]; LandingHeight input double; cutIntXY input double; eI_prec input single; eI output single
function [Torques, eR, Omega_ref, Iterm, Dterm, GyroTerm, eI] = AttitudeController(Q_ref, Q_est, Omega_est, I, Komega_perso, Ktorques_perso, Kint_perso, dt, Pos, LandingHeight, cutIntXY, eI_prec)
    
    % calculate the Attitude error 
    Q_tilde = QuaternionProduct(InvQuaternion(Q_est), Q_ref);
%     s_tilde = 2*acos(Q_tilde(1));
%     v_tilde = Q_tilde(2:4)/sin(s_tilde/2);
    s_tilde = Q_tilde(1);
    v_tilde = Q_tilde(2:4);
    eR = s_tilde*v_tilde;
    
    if s_tilde >= 0
        Omega_ref = 2*diag(Komega_perso)*v_tilde;
    else
        Omega_ref = -2*diag(Komega_perso)*v_tilde;
    end
    
    eI = eI_prec;
    if Pos(3)>= LandingHeight && cutIntXY == 0
        eI = eI_prec + Kint_perso.*(eR*dt);
    elseif Pos(3)>= LandingHeight && cutIntXY == 1
        eI(1:2) = eI_prec(1:2);
        eI(3) = eI_prec(3) + Kint_perso(3).*(eR(3)*dt);
    end
    
    Dterm = I*diag(Ktorques_perso)*(Omega_ref-Omega_est);
    Iterm = I*eI;
    
    GyroTerm = single([0 0 0]'); % cross(Omega_est, I*Omega_est);
    
    Torques = Dterm + Iterm + GyroTerm;
end

== matlab function GUMSTIX/Torques Disturbances/Triggered Subsystem1/MATLAB Function ==
  data: TorquesDistMag input single; TorquesDist output single; Time input single; Dt input single
function TorquesDist = fcn(TorquesDistMag, Time, Dt)

    %#codegen
    
    TorquesDist = single(zeros(3,1));

    t1 = single(1);
    t2 = single(5);
    t3 = single(9);

    if (Time>=t1 && Time<t1+Dt)
        TorquesDist(1) = TorquesDistMag(1);
    elseif (Time>=t2 && Time<t2+Dt)
        TorquesDist(2) = TorquesDistMag(2);
    elseif (Time>=t3 && Time<t3+Dt)
        TorquesDist(3) = TorquesDistMag(3);
    else
        % do nothing, all torques are null
    end

end

== matlab function GUMSTIX/Attitude controller/CTL_ATT_NL/Euler 2 Quaternion1 ==
  data: angles input double; Q output double
function Q  = Euler2Quaternion(angles)
    
    Q = Euler2Quaternion(angles(1), angles(2), angles(3));

end

== matlab function GUMSTIX/Arena Security/MATLAB Function ==
  data: xyz input double size=3; secu_ON output double; PositionSecuMin parameter double size=3; PositionSecuMax parameter double size=3
function secu_ON = fcn(xyz, PositionSecuMin, PositionSecuMax)
%#codegen

x = xyz(1);
y = xyz(2);
z = xyz(3);

if ( x >= PositionSecuMax(1) || x <= PositionSecuMin(1) ||  y >= PositionSecuMax(2) || y <= PositionSecuMin(2) ||  z >= PositionSecuMax(3) || z <= PositionSecuMin(3) )
    secu_ON = 1;
else
    secu_ON = 0;
end

end

== matlab function GUMSTIX/Attitude controller/CTL_ATT_NL/Angles Disturbances/Triggered Subsystem/MATLAB Function ==
  data: AnglesDistMag input single; AnglesDist output single; Time input single; Dt input single
function AnglesDist = fcn(AnglesDistMag, Time, Dt)

    %#codegen
    
    AnglesDist = single(zeros(3,1));

    t1 = single(1);
    t2 = single(5);
    t3 = single(9);
    
    Dt = Dt/2;

    if (Time>=t1 && Time<t1+Dt)
        AnglesDist(1) = AnglesDistMag(1);
    elseif (Time>=t1+Dt && Time<t1+2*Dt)
        AnglesDist(1) = -AnglesDistMag(1);
    elseif (Time>=t2 && Time<t2+Dt)
        AnglesDist(2) = AnglesDistMag(2);
    elseif (Time>=t2+Dt && Time<t2+2*Dt)
        AnglesDist(2) = -AnglesDistMag(2);
    elseif (Time>=t3 && Time<t3+Dt)
        AnglesDist(3) = AnglesDistMag(3);
    elseif (Time>=t3+Dt && Time<t3+2*Dt)
        AnglesDist(3) = -AnglesDistMag(3);
    else
        % do nothing, all torques are null
    end

end

== matlab function GUMSTIX/Control Mix/Control_mix/Mixage ==
  data: iGamma input double; ThrustTorques input double; gamma input double; omega2 output double
function omega2 = mixage(iGamma,ThrustTorques,gamma)
% Inverse Gamma matrix
% INPUTS
%	- gamma :	folding angle		[deg]
% OUTPUTS
%	- omega2:	Rotor speed square	[rad]^2

omega2 = iGamma(:,:,gamma+1)*ThrustTorques;
		
end

== matlab function GUMSTIX/Torques saturation/MATLAB Function ==
  data: TorquesSat input double; gamma input double; TSat output double
function TSat = torque_select(TorquesSat,gamma)
% Select torque saturation (depends of gamma)

TSat = TorquesSat(:,gamma+1);

end

== matlab function GUMSTIX/ESTIMATOR/Quaternion 2 Euler ==
  data: Q_hat input double; phi_hat output double; theta_hat output double; psi_hat output double
function [phi_hat, theta_hat, psi_hat] = rot2rad(Q_hat)
    
    %#codegen
    
    [phi_hat, theta_hat, psi_hat] = Quaternion2Euler(Q_hat);

end

== matlab function GUMSTIX/Positioning Mode/Euler 2 Quaternion1 ==
  data: angles input double; Q output double
function Q  = Euler2Quaternion(angles)
    
    %#codegen
    Q = Euler2Quaternion(angles(1), angles(2), angles(3));

end
